simulink subsystem "HIL_Receive_TCP_Data"  (R2022b)
settings: Solver=VariableStepAuto  StartTime=0.0  StopTime=10.0  RelTol=1e-3
model mask{mi_ip=0, mi_port=0, f=0}
  mask prompts: mi_ip "Server IP"; mi_port "Server PORT"; f "Sampling Frequency"
libraries: slrealtimeiplib x2
settings Model: Creator=ramuj  LastModifiedBy=ramuj

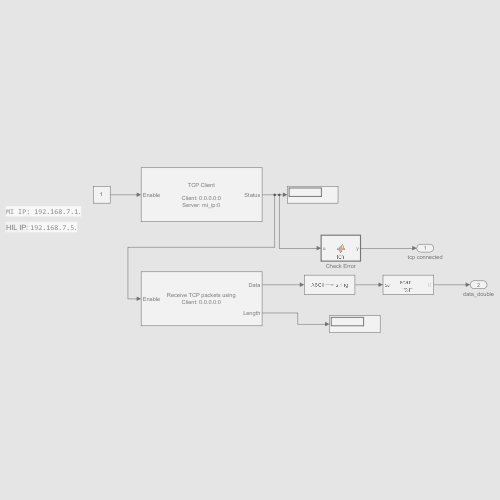
[thumbnail: Simulink's stored preview of the top-level diagram]
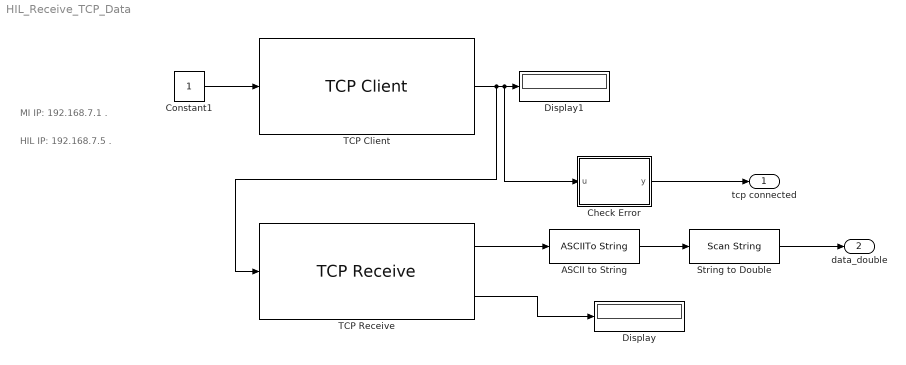
== system HIL_Receive_TCP_Data ==
  note: MI IP: 192.168.7.1 .
  note: HIL IP: 192.168.7.5 .
  ASCII to String : ASCIIToString
  Check Error : MATLAB Function  TreatAsAtomicUnit=on
  Constant1 : Constant
  Display : Display
  Display1 : Display
  String to Double : ScanString  Format="\"%lf\""
  TCP Client : slrealtimeiplib/TCP Client  Priority=-1  useHostTargetConn=off  remoteAddress=mi_ip  remotePort=mi_port
  TCP Receive : slrealtimeiplib/TCP Receive  socketAddPortVal=Client: 0.0.0.0:0  rcvWidth=16  sampleTime=1/f
  tcp connected : Outport
  data_double : Outport  Port=2
  wires:
  Constant1/1 -> TCP Client/1
  TCP Client/1 -> TCP Receive/1, Display1/1, Check Error/1(u)
  Check Error/1(y) -> tcp connected/1
  ASCII to String/1 -> String to Double/1
  String to Double/1 -> data_double/1
  TCP Receive/1 -> ASCII to String/1
  TCP Receive/2 -> Display/1

== matlab function HIL_Receive_TCP_Data/Check Error ==
  data: u input; y output
function y = fcn(u)

    if(u == 1)
        y = "Connected";
    else 
        y = "Error";
    end
end
